simulink model "es_VI_1_2"  (Simulink 7.0)
settings: Solver=ode45  StartTime=0.0  StopTime=40.0  RelTol=1e-5
values from neighbouring files (symbols this model uses):
  Kc = 800    [es_VI_1.m]    (also in es_VI_2.m = -0.1)
  Kr = 2    [es_VI_1.m]    (also in es_VI_2.m = 0.5)
libraries: cstblocks x1, simulink x1
settings Model: Creator=Indri  LastModifiedBy=Indri  ExtModeTrigMode=oneshot  ExtModeArmWhenConnect=off
settings DataIOCC: LimitDataPoints=off
settings OptimizationCC: BlockReduction=off  BooleanDataType=off
settings DebuggingCC: SaveWithParameterizedLinksMsg=none  SignalResolutionControl=TryResolveAllWithWarning  SolverPrmCheckMsg=none  MultiTaskDSMMsg=warning  MultiTaskCondExecSysMsg=none  StrictBusMsg=None
settings HardwareCC: TargetUnknown=on
settings RTWCC: IncludeERTFirstTime=on

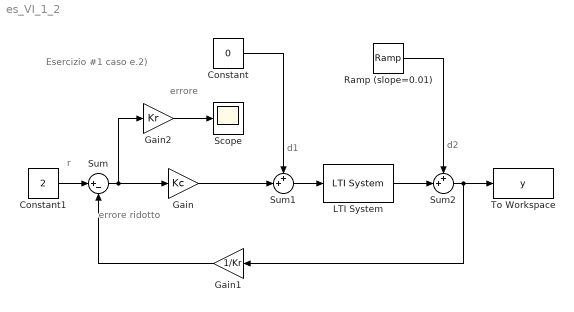
== system es_VI_1_2 ==
  note: errore
      | ridotto
  note: errore
  note: Esercizio #1
      | caso e.2)
  note: r
  note: d1
  note: d2
  Constant : Constant  Value=0
  Constant1 : Constant  Value=2
  Gain : Gain  Gain=Kc  SaturateOnIntegerOverflow=on
  Gain1 : Gain  Orientation=left  Gain=1/Kr  SaturateOnIntegerOverflow=on
  Gain2 : Gain  Gain=Kr  SaturateOnIntegerOverflow=on
  LTI System : cstblocks/LTI System  SystemSampleTime=-1  sys=F  IC=[]
  Ramp (slope=0.01) : simulink/Sources/Ramp  SystemSampleTime=-1  slope=0.01  start=0  X0=0
  Scope : Scope
  Sum : Sum  Inputs=|+-  SaturateOnIntegerOverflow=on  InputSameDT=on
  Sum1 : Sum  Inputs=++|  SaturateOnIntegerOverflow=on  InputSameDT=on
  Sum2 : Sum  Inputs=++|  SaturateOnIntegerOverflow=on  InputSameDT=on
  To Workspace : ToWorkspace  VariableName=y  SampleTime=-1  SaveFormat=Array
  wires:
  Constant1/1 -> Sum/1
  Gain/1 -> Sum1/2
  Gain1/1 -> Sum/2
  Sum/1 -> Gain/1, Gain2/1
  Gain2/1 -> Scope/1
  Constant/1 -> Sum1/1
  Sum1/1 -> LTI System/1
  LTI System/1 -> Sum2/2
  Sum2/1 -> To Workspace/1, Gain1/1
  Ramp (slope=0.01)/1 -> Sum2/1
